simulink model "firstModel"  (R2023a)
settings: Solver=FixedStepAuto  StartTime=0.0  StopTime=inf  FixedStep=10e-3  RelTol=1e-3  EnableMultiTasking=on
libraries: arduinolib x12, simulink x4, arduinosensorlib x4, slpidlib x1
settings Model: ExtModeTrigDuration=2  Creator=tolla  LastModifiedBy=tolla
settings OptimizationCC: EnhancedBackFolding=on  PassReuseOutputArgsThreshold=0  MaxStackSize=64  OptimizeBlockOrder=speed  DifferentSizesBufferReuse=on  OptimizationCustomize=off
settings DebuggingCC: ParameterTunabilityLossMsg=error
settings HardwareCC: ProdBitPerPointer=32  ProdBitPerSizeT=32  ProdBitPerPtrDiffT=32  ProdLargestAtomicInteger=Long  ProdLargestAtomicFloat=Double  ProdWordSize=32  ProdHWDeviceType=ARM Compatible->ARM Cortex  UseEmbeddedCoderFeatures=off
settings SFSimCC: MATLABDynamicMemAlloc=off
settings RTWCC: Description=Embedded Coder  SystemTargetFile=ert.tlc  HardwareBoard=ESP32-WROOM(Arduino Compatible)  TLCOptions="-aInlineSetEventsForThisBaseRateFcn=TLC_FALSE -aSuppressMultiTaskScheduler=TLC_FALSE  -aRateBasedStepFcn=0"  TemplateMakefile=ert_default_tmf  Toolchain=ESP32  BuildConfiguration=Faster Runs
settings CodeAppCC: ForceParamTrailComments=on  OperatorAnnotations=on
settings ERTTargetCC: ERTCustomFileBanners=off  SupportContinuousTime=on  SupportNonInlinedSFcns=on  RemoveResetFunc=off  SupportVariableSizeSignals=on  ModelStepFunctionPrototypeControlCompliant=off  ExtModeTransport=3  ExtModeStaticAlloc=on  ExtModeAutomaticAllocSize=off  ExtModeStaticAllocSize=65536  ExtModeMexFile=ext_xcp  ExtModeIntrfLevel=Level2 - Open

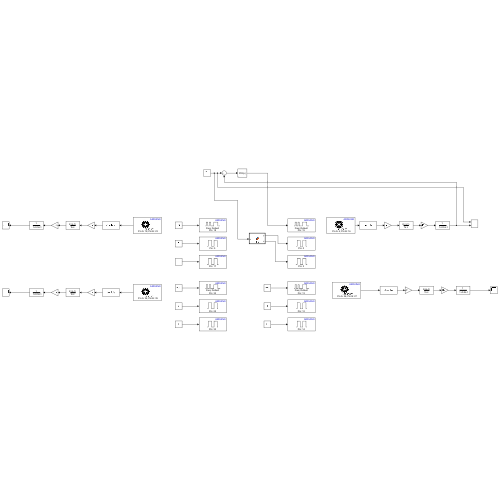
[thumbnail: Simulink's stored preview of the top-level diagram]
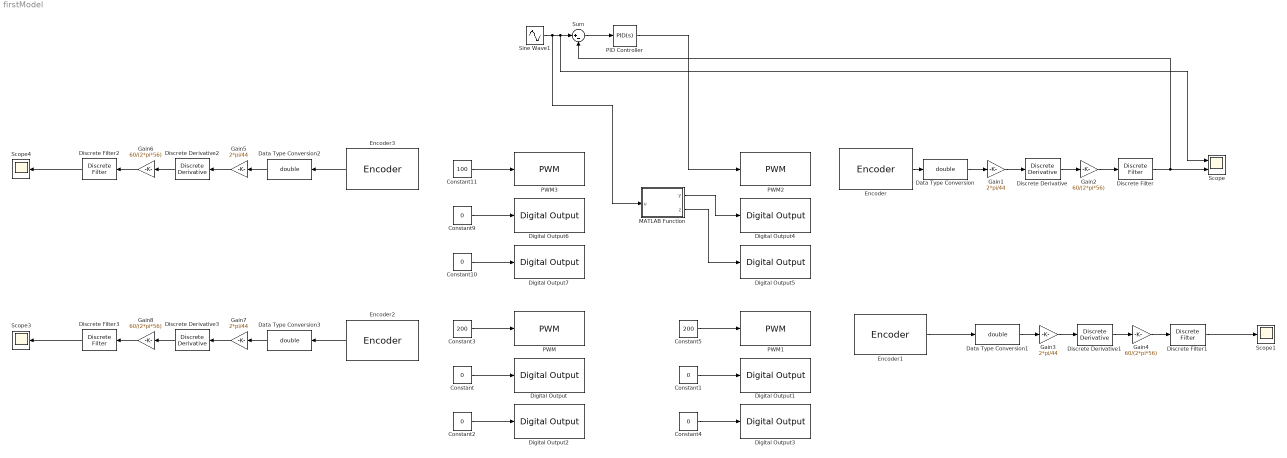
== system firstModel ==
  Constant{,1..2,4,9..10} (6 alike) : Constant  Value=0
  Constant11 : Constant  Value=100
  Constant3 : Constant  Value=200
  Constant5 : Constant  Value=200
  Data Type Conversion{,1..3} (4 alike) : DataTypeConversion  OutDataTypeStr=double  SaturateOnIntegerOverflow=off  RndMeth=Floor
  Digital Output : arduinolib/Digital Output  pinNumber=25  Direction=output  blockPlatform=arduino
  Digital Output1 : arduinolib/Digital Output  pinNumber=12  Direction=output  blockPlatform=arduino
  Digital Output2 : arduinolib/Digital Output  pinNumber=33  Direction=output  blockPlatform=arduino
  Digital Output3 : arduinolib/Digital Output  pinNumber=14  Direction=output  blockPlatform=arduino
  Digital Output4 : arduinolib/Digital Output  pinNumber=0  Direction=output  blockPlatform=arduino
  Digital Output5 : arduinolib/Digital Output  pinNumber=2  Direction=output  blockPlatform=arduino
  Digital Output6 : arduinolib/Digital Output  pinNumber=5  Direction=output  blockPlatform=arduino
  Digital Output7 : arduinolib/Digital Output  pinNumber=17  Direction=output  blockPlatform=arduino
  Discrete Derivative{,1..3} (4 alike) : simulink/Discrete/Discrete Derivative  gainval=1.0  ICPrevScaledInput=0.0  OutMin=[]  OutMax=[]  OutDataType=fixdt(1, 16)  OutScaling=2^-10  DoSatur=off
  Discrete Filter{,1..3} (4 alike) : DiscreteFilter
  Encoder : arduinosensorlib/Encoder  InputA=4  InputB=16  Mode=No reset  SampleTime=-1
  Encoder1 : arduinosensorlib/Encoder  InputA=26  InputB=27  Mode=No reset  SampleTime=-1
  Encoder2 : arduinosensorlib/Encoder  InputA=34  InputB=35  Mode=No reset  SampleTime=-1
  Encoder3 : arduinosensorlib/Encoder  InputA=19  InputB=23  Mode=No reset  SampleTime=-1
  Gain{1,3,5,7} (4 alike) : Gain  Gain=2*pi/44
  Gain{2,4,6,8} (4 alike) : Gain  Gain=60/(2*pi*56)
  MATLAB Function : MATLAB Function  TreatAsAtomicUnit=on
  PID Controller : slpidlib/PID Controller  Controller=PID  Form=Parallel  TimeDomain=Continuous-time  UseExternalTs=off  SampleTime=-1  IntegratorMethod=Forward Euler  FilterMethod=Forward Euler  ControllerParametersSource=internal  P=20  I=0  UseKiTs=off  D=0  N=100  UseFilter=on  TunerSelectOption=Transfer Function Based (PID Tuner App)  InitialConditionSource=internal  InitialConditionForIntegrator=0  InitialConditionForFilter=0  DifferentiatorICPrevScaledInput=0  ExternalReset=none  TrackingMode=off  Kt=1  LimitOutput=off  SatLimitsSource=internal  UpperSaturationLimit=inf  LowerSaturationLimit=-inf  LinearizeAsGain=on  AntiWindupMode=none  Kb=1  LimitIntegrator=off  UpperIntegratorSaturationLimit=inf  LowerIntegratorSaturationLimit=-inf  POutMin=[]  POutMax=[]  IOutMin=[]  IOutMax=[]  DOutMin=[]  DOutMax=[]  NOutMin=[]  NOutMax=[]  SumOutMin=[]  SumOutMax=[]  SaturationOutMin=[]  SaturationOutMax=[]  PParamMin=[]  PParamMax=[]  IParamMin=[]  IParamMax=[]  DParamMin=[]  DParamMax=[]  NParamMin=[]  NParamMax=[]  KbParamMin=[]  KbParamMax=[]  KtParamMin=[]  KtParamMax=[]  KbOutMin=[]  KbOutMax=[]  KtOutMin=[]  KtOutMax=[]  IntegratorOutMin=[]  IntegratorOutMax=[]  FilterOutMin=[]  FilterOutMax=[]  SumI1OutMin=[]  SumI1OutMax=[]  SumI2OutMin=[]  SumI2OutMax=[]  SumI3OutMin=[]  SumI3OutMax=[]  SumI4OutMin=[]  SumI4OutMax=[]  SumDOutMin=[]  SumDOutMax=[]  DifferentiatorOutMin=[]  DifferentiatorOutMax=[]  FilterDiffOutCoefMin=[]  FilterDiffOutCoefMax=[]  ReciprocalOutMin=[]  ReciprocalOutMax=[]  SumDenOutMin=[]  SumDenOutMax=[]  SumNumOutMin=[]  SumNumOutMax=[]  DivideOutMin=[]  DivideOutMax=[]  UdiffTsProdOutMin=[]  UdiffTsProdOutMax=[]  NTsProdOutMin=[]  NTsProdOutMax=[]  UintegralTsProdOutMin=[]  UintegralTsProdOutMax=[]  UngainTsProdOutMin=[]  UngainTsProdOutMax=[]  ClampingZeroOutDataTypeStr=Inherit: Inherit via back propagation  ClampingZeroOutMin=[]  ClampingZeroOutMax=[]  FilterDenConstantOutDataTypeStr=Inherit: Inherit via back propagation  FilterDenConstantOutMin=[]  FilterDenConstantOutMax=[]  PCopyOutDataTypeStr=Inherit: Inherit via back propagation  PCopyOutMin=[]  PCopyOutMax=[]  NCopyOutDataTypeStr=Inherit: Inherit via back propagation  NCopyOutMin=[]  NCopyOutMax=[]  IntegratorContinuousStateAttributes=''  IntegratorStateMustResolveToSignalObject=off  IntegratorRTWStateStorageClass=Auto  FilterContinuousStateAttributes=''  FilterStateMustResolveToSignalObject=off  FilterRTWStateStorageClass=Auto  ParallelPVariant=InternalParameters  IdealPVariant=Disabled  IVariant=InternalParameters  DVariant=InternalParameters  IntegratorVariant=Continuous  SatVariant=Disabled  AWVariant=Passthrough  PCopyVariant=Disabled  TRVariant=Disabled  FdbkBlocksVariant=Forward  IdealPFdbkVariant=Disabled  SatFdbkVariant=Disabled  DerivativeFilterVariant=ContFilter  NVariant=InternalParameters  NCopyVariant=Disabled  FilterICVariant=InternalICsFilter  IntegratorICVariant=InternalICs  ExternalResetVariant=Disabled  TRSumVariant=Passthrough  SumFdbkVariant=Disabled  SumVariant=Sum_PID  TsampFilterVariant=InternalTs  TsampNgainVariant=Passthrough  TsampIntegralVariant=Disabled_SignalSpec  ExternalSaturationOutDataTypeStr=Inherit: Same as second input
  PWM : arduinolib/PWM  pinNumber=32  frequencyType=Default  desiredFrequency=490.2  achievableFrequency=490.2
  PWM1 : arduinolib/PWM  pinNumber=13  frequencyType=Default  desiredFrequency=490.2  achievableFrequency=490.2
  PWM2 : arduinolib/PWM  pinNumber=15  frequencyType=Default  desiredFrequency=490.2  achievableFrequency=490.2
  PWM3 : arduinolib/PWM  pinNumber=18  frequencyType=Default  desiredFrequency=490.2  achievableFrequency=490.2
  Scope : Scope  NumInputPorts=2
  Scope1 : Scope
  Scope3 : Scope
  Scope4 : Scope
  Sine Wave1 : Sin  Amplitude=75  Frequency=2*pi/5  SampleTime=0
  Sum : Sum  Inputs=|+-
  wires:
  Constant/1 -> Digital Output/1
  Constant2/1 -> Digital Output2/1
  Constant3/1 -> PWM/1
  Constant4/1 -> Digital Output3/1
  Constant1/1 -> Digital Output1/1
  Constant5/1 -> PWM1/1
  MATLAB Function/2(z) -> Digital Output5/1
  MATLAB Function/1(y) -> Digital Output4/1
  Constant10/1 -> Digital Output7/1
  Constant9/1 -> Digital Output6/1
  Constant11/1 -> PWM3/1
  Encoder2/1 -> Data Type Conversion3/1
  Encoder3/1 -> Data Type Conversion2/1
  Encoder/1 -> Data Type Conversion/1
  Discrete Derivative/1 -> Gain2/1
  Data Type Conversion/1 -> Gain1/1
  Gain1/1 -> Discrete Derivative/1
  Gain2/1 -> Discrete Filter/1
  PID Controller/1 -> PWM2/1
  Gain4/1 -> Discrete Filter1/1
  Gain3/1 -> Discrete Derivative1/1
  Discrete Filter1/1 -> Scope1/1
  Discrete Derivative1/1 -> Gain4/1
  Data Type Conversion1/1 -> Gain3/1
  Encoder1/1 -> Data Type Conversion1/1
  Gain6/1 -> Discrete Filter2/1
  Gain5/1 -> Discrete Derivative2/1
  Discrete Filter2/1 -> Scope4/1
  Discrete Derivative2/1 -> Gain6/1
  Data Type Conversion2/1 -> Gain5/1
  Data Type Conversion3/1 -> Gain7/1
  Discrete Filter3/1 -> Scope3/1
  Discrete Derivative3/1 -> Gain8/1
  Gain8/1 -> Discrete Filter3/1
  Gain7/1 -> Discrete Derivative3/1
  Sine Wave1/1 -> MATLAB Function/1(u), Scope/1, Sum/1
  Sum/1 -> PID Controller/1
  Discrete Filter/1 -> Scope/2, Sum/2

== matlab function firstModel/MATLAB Function ==
  data: u input; y output; z output
function [y,z] = fcn(u)
if u > 0
     y = 1;
     z = 0;
end
if u < 0 
    y = 0;
    z = 1;
end
